simulink model "tether002_th"  (R2020a)
settings: Solver=VariableStepAuto  StartTime=0.0  StopTime=simTime  RelTol=1e-3
values from neighbouring files (symbols this model uses):
  linkFlowVelVecs = [10*ones(1,numNodes-1);10*ones(1,numNodes-1);.001*ones(1,numNodes-1)]    [tether002_ts.m]
  OriginalLengths = [((TetherLength-TopLinkLength)/(numNodes-2))*ones(1,numNodes-2),TopLinkLength]    [tether002_ts.m]
  ReelInVel = -(LengthI-LengthF)/simTime    (= -0.099)    [tether002_ts.m]
  TetherLength = 100    [tether002_ts.m]
libraries: tether002_ul x1
settings Model: Creator=mitch  LastModifiedBy=mr-jo

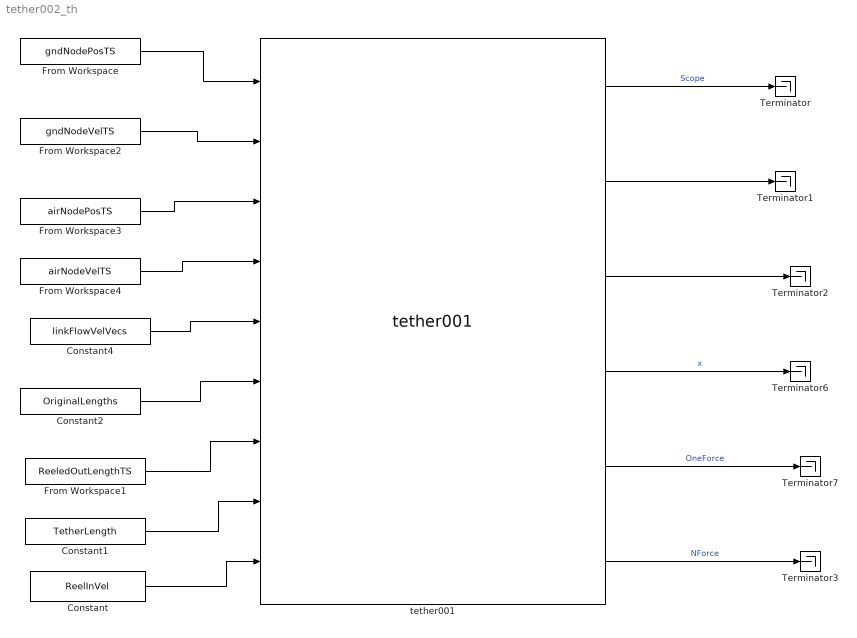
== system tether002_th ==
  Constant : Constant  Value=ReelInVel
  Constant1 : Constant  Value=TetherLength
  Constant2 : Constant  Value=OriginalLengths
  Constant4 : Constant  Value=linkFlowVelVecs
  From Workspace : FromWorkspace  VariableName=gndNodePosTS
  From Workspace1 : FromWorkspace  VariableName=ReeledOutLengthTS  Interpolate=off  OutputAfterFinalValue=Holding final value
  From Workspace2 : FromWorkspace  VariableName=gndNodeVelTS
  From Workspace3 : FromWorkspace  VariableName=airNodePosTS
  From Workspace4 : FromWorkspace  VariableName=airNodeVelTS
  Terminator{,1..3,6..7} (6 alike) : Terminator
  tether001 : tether002_ul/tether001  SystemSampleTime=-1  Latency=0  AutoFrameSizeCalculation=off
  wires:
  From Workspace/1 -> tether001/1
  From Workspace2/1 -> tether001/2
  From Workspace3/1 -> tether001/3
  From Workspace4/1 -> tether001/4
  Constant4/1 -> tether001/5
  Constant2/1 -> tether001/6
  From Workspace1/1 -> tether001/7
  Constant1/1 -> tether001/8
  Constant/1 -> tether001/9
  tether001/1 -> Terminator/1  "Scope"
  tether001/2 -> Terminator1/1
  tether001/3 -> Terminator2/1
  tether001/4 -> Terminator6/1  "x"
  tether001/6 -> Terminator3/1  "NForce"
  tether001/5 -> Terminator7/1  "OneForce"
